simulink model "backstepping"  (R2022b)
settings: Solver=VariableStepAuto  StartTime=0.0  StopTime=30.0  RelTol=1e-3
values from neighbouring files (symbols this model uses):
  Lamda = 10*eye(3)    [init.m]
settings Model: Creator=alexi  LastModifiedBy=alexi

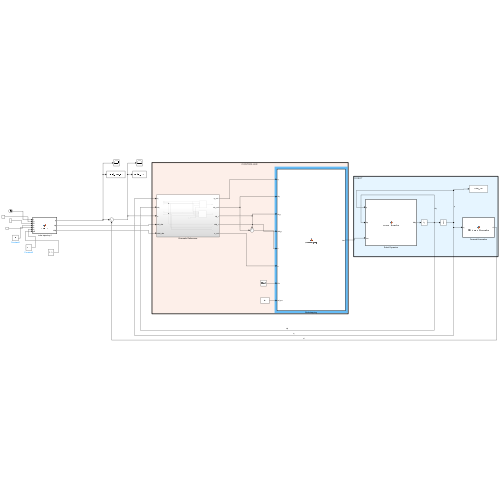
[thumbnail: Simulink's stored preview of the top-level diagram]
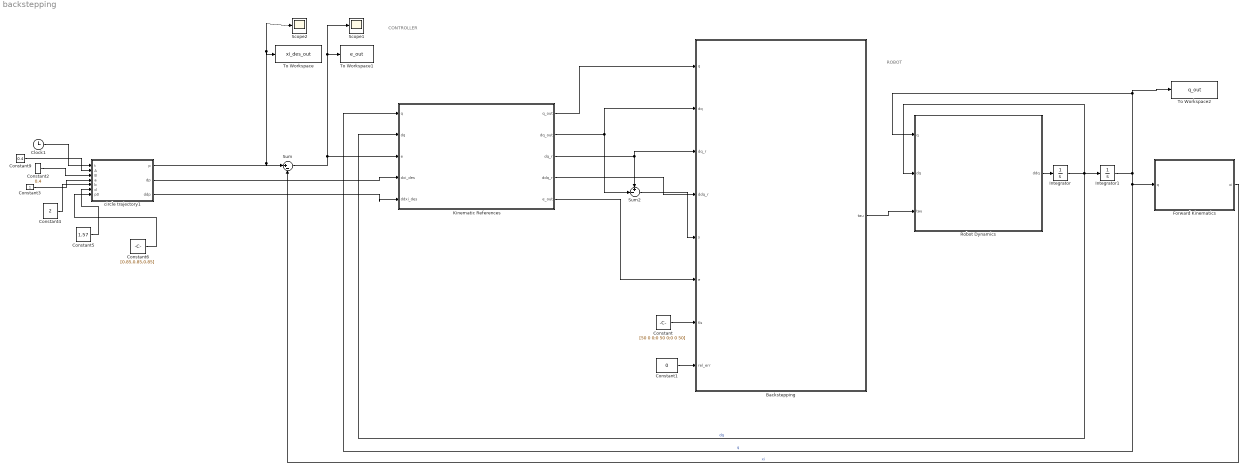
== system backstepping ==
  note: CONTROLLER
  note: ROBOT
  Backstepping : MATLAB Function  TreatAsAtomicUnit=on
  Clock1 : Clock
  Constant : Constant  Value=[50 0 0;0 50 0;0 0 50]
  Constant1 : Constant  Value=0
  Constant2 : Constant  Value=0.4
  Constant3 : Constant
  Constant4 : Constant  Value=2
  Constant5 : Constant  Value=1.57
  Constant6 : Constant  Value=[0.85,0.85,0.85]
  Constant9 : Constant  Value=0.4
  Forward Kinematics : MATLAB Function  TreatAsAtomicUnit=on
  Integrator : Integrator  InitialCondition=[0,0,0]'
  Integrator1 : Integrator  InitialCondition=[0.25,0.25,0.25]'
  Kinematic References : Subsystem
  Robot Dynamics : MATLAB Function  TreatAsAtomicUnit=on
  Scope1 : Scope
  Scope2 : Scope
  Sum : Sum  Inputs=|+-
  Sum2 : Sum  Inputs=+-|
  To Workspace : ToWorkspace  VariableName=xi_des_out  SaveFormat=Timeseries  SampleTime=-1
  To Workspace1 : ToWorkspace  VariableName=e_out  SaveFormat=Timeseries  SampleTime=-1
  To Workspace2 : ToWorkspace  VariableName=q_out  SaveFormat=Timeseries  SampleTime=-1
  circle trajectory1 : MATLAB Function  TreatAsAtomicUnit=on
  wires:
  Kinematic References/4(ddq_r) -> Backstepping/4(ddq_r)
  circle trajectory1/1(p) -> Scope2/1, To Workspace/1, Sum/1
  Kinematic References/2(dq_out) -> Sum2/2, Backstepping/2(dq)
  Sum2/1 -> Backstepping/5(s)
  circle trajectory1/3(ddp) -> Kinematic References/5(ddxi_des)
  Constant/1 -> Backstepping/7(Ks)
  Forward Kinematics/1(xi) -> Sum/2  "xi"
  Kinematic References/1("q_out ") -> Backstepping/1(q)
  Integrator/1 -> Robot Dynamics/2(dq), Kinematic References/2(dq), Integrator1/1  "dq"
  Sum/1 -> Kinematic References/3(e), To Workspace1/1, Scope1/1
  Integrator1/1 -> Kinematic References/1(q), Forward Kinematics/1(q), To Workspace2/1, Robot Dynamics/1(q)  "q"
  circle trajectory1/2(dp) -> Kinematic References/4(dxi_des)
  Backstepping/1(tau) -> Robot Dynamics/3(tau)
  Robot Dynamics/1(ddq) -> Integrator/1
  Kinematic References/3(dq_r) -> Backstepping/3(dq_r), Sum2/1
  Kinematic References/5(e_out) -> Backstepping/6(e)
  Clock1/1 -> circle trajectory1/1(t)
  Constant1/1 -> Backstepping/8(rel_err)
  Constant9/1 -> circle trajectory1/2(A)
  Constant2/1 -> circle trajectory1/3(B)
  Constant3/1 -> circle trajectory1/4(a)
  Constant4/1 -> circle trajectory1/5(b)
  Constant5/1 -> circle trajectory1/6(d)
  Constant6/1 -> circle trajectory1/7(p0)

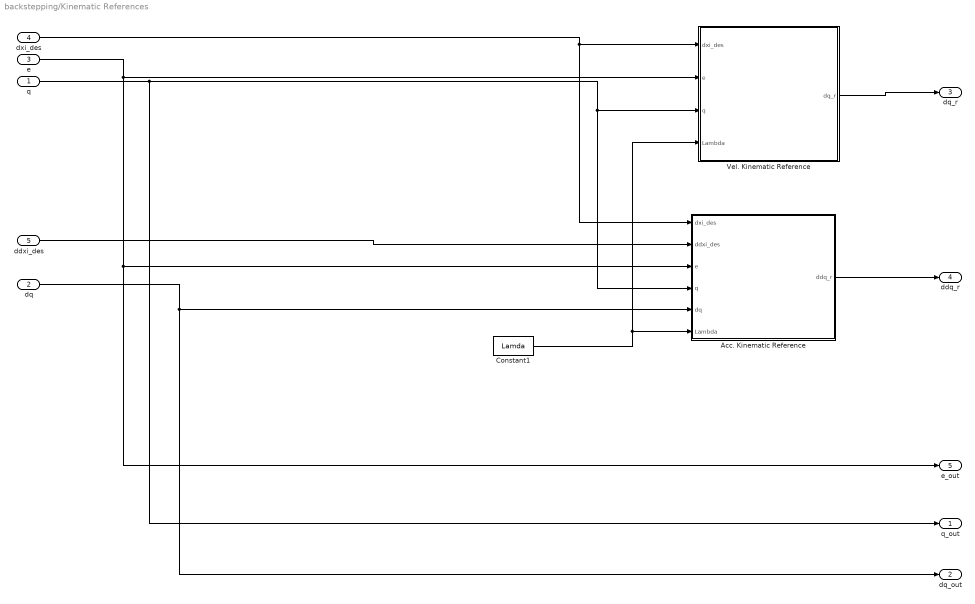
== system backstepping/Kinematic References ==
  q : Inport
  dq : Inport  Port=2
  e : Inport  Port=3
  dxi_des : Inport  Port=4
  ddxi_des : Inport  Port=5
  Acc. Kinematic Reference : MATLAB Function  TreatAsAtomicUnit=on
  Constant1 : Constant  Value=Lamda
  "Vel. Kinematic Reference " : MATLAB Function  TreatAsAtomicUnit=on
  "q_out " : Outport  VectorParamsAs1DForOutWhenUnconnected=off
  dq_out : Outport  Port=2  VectorParamsAs1DForOutWhenUnconnected=off
  dq_r : Outport  Port=3  VectorParamsAs1DForOutWhenUnconnected=off
  ddq_r : Outport  Port=4  VectorParamsAs1DForOutWhenUnconnected=off
  e_out : Outport  Port=5  VectorParamsAs1DForOutWhenUnconnected=off
  wires:
  ddxi_des/1 -> Acc. Kinematic Reference/2(ddxi_des)
  e/1 -> e_out/1, Acc. Kinematic Reference/3(e), "Vel. Kinematic Reference "/2(e)
  dxi_des/1 -> Acc. Kinematic Reference/1(dxi_des), "Vel. Kinematic Reference "/1(dxi_des)
  Constant1/1 -> "Vel. Kinematic Reference "/4(Lambda), Acc. Kinematic Reference/6(Lambda)
  "Vel. Kinematic Reference "/1(dq_r) -> dq_r/1
  dq/1 -> dq_out/1, Acc. Kinematic Reference/5(dq)
  q/1 -> "q_out "/1, Acc. Kinematic Reference/4(q), "Vel. Kinematic Reference "/3(q)
  Acc. Kinematic Reference/1(ddq_r) -> ddq_r/1

== matlab function backstepping/Kinematic References/Acc. Kinematic Reference ==
  data: dxi_des input; ddq_r output; ddxi_des input; e input; q input; dq input; Lambda input
function ddq_r = acc_kinematic_reference(dxi_des, ddxi_des, e, q, dq, Lambda)

coder.extrinsic('disp');

J = zeros(3,3);
dJ = zeros(3,3);

dq1 = dq(1);
dq2 = dq(2);
dq3 = dq(3);

q1 = q(1);
q2 = q(2);
q3 = q(3);

a1 = 1;
a2 = 1;
a3 = 1;

% Computing jacobian and derivative
J = [- a1*sin(q1) - a3*cos(q3)*(cos(q1)*sin(q2) + cos(q2)*sin(q1)) - a2*cos(q1)*sin(q2) - a2*cos(q2)*sin(q1), -a3*cos(q3)*(cos(q1)*sin(q2) +cos(q2)*sin(q1)) - a2*cos(q1)*sin(q2) - a2*cos(q2)*sin(q1), -a3*sin(q3)*(cos(q1)*cos(q2) - sin(q1)*sin(q2)); ...
    a1*cos(q1) + a3*cos(q3)*(cos(q1)*cos(q2) - sin(q1)*sin(q2)) + a2*cos(q1)*cos(q2) - a2*sin(q1)*sin(q2),   a3*cos(q3)*(cos(q1)*cos(q2) - sin(q1)*sin(q2)) + a2*cos(q1)*cos(q2) - a2*sin(q1)*sin(q2),  -a3*sin(q3)*(cos(q1)*sin(q2) + cos(q2)*sin(q1)); ...
    0,0,- a3*cos(q3)*(cos(q1)*sin(q2) + cos(q2)*sin(q1))^2 - a3*cos(q3)*(cos(q1)*cos(q2) - sin(q1)*sin(q2))^2];

a11 = -a1*dq1*cos(q1)-a3*(dq1*cos(q1+q2)+ dq2*cos(q1+q2))*sin(q3)-a2*(dq1*cos(q1+q2)+ dq2*cos(q1+q2));
a12 = -a3*( dq1*cos(q1+q2)+ dq2*cos(q1+q2))*sin(q3)-a2*( dq1*cos(q1+q2)+ dq2*cos(q1+q2));
a13 = -a3*( dq1*cos(q1+q2)+ dq2*cos(q1+q2))*cos(q3);
a21 = -a1*dq1*sin(q1)-a3*( dq1*sin(q1+q2)+ dq2*sin(q1+q2))*cos(q3)-a2*( dq1*sin(q1+q2)+ dq2*sin(q1+q2));
a22 = -a3*(dq1*sin(q1+q2)+dq2*sin(q1+q2))*sin(q3)-a2*(dq1*sin(q1+q2)+dq2*sin(q1+q2));
a23 = -a3*(dq1*cos(q1+q2)+dq2*cos(q1+q2))*sin(q3);
a31 = 0;
a32 = 0;
a33 = 2*a3*(dq1*cos(q1+q2)+dq2*cos(q1+q2))*sin(q1+q2)*sin(q3)-2*a3*(dq1*sin(q1+q2)+dq2*sin(q1+q2))*cos(q1+q2)*sin(q3);

dJ = [a11,a12,a13;a21,a22,a23;a31,a32,a33];

ddq_r = inv(J) * (ddxi_des + Lambda*dxi_des - Lambda*J*dq) ...
- inv(J)*dJ*inv(J)*(dxi_des + Lambda*e);
end

== matlab function backstepping/circle trajectory1 ==
  data: t input; p output; dp output; ddp output; A input; B input; a input; b input; d input; p0 input
function [p,dp,ddp] = lissajous(t,A,B,a,b,d,p0)
C = 0.1;  % Ampiezza dell'oscillazione in z
c = 0.2;  % Frequenza in z
phi = pi/4;
p = [A*sin(a*t+d); B*sin(b*t);C*sin(c*t + phi)] + p0;
dp = [A*a*cos(a*t+d); B*b*cos(b*t);C*c*cos(c*t+phi)];
ddp = [-A*a^2*sin(a*t+d); -B*b^2*sin(b*t);-C*c^2*sin(c*t+phi)];
% a = 0.2;    % Ampiezza lungo l'asse X
% b = 0.2;    % Ampiezza lungo l'asse Y
% p0 = [1;0.8;0.8];
% 
% x = a * cos(t);
% y = b * sin(t);
% z =  0.1 * sin(t);
% 
% p = [x y z]'+p0;
% 
% dx = -a*sin(t);
% dy = b*cos(t);
% dz = 0.5*cos(t);
% 
% dp = [dx dy dz]';
% 
% ddx = -a*cos(t);
% ddy = -b*sin(t);
% ddz = -0.5*sin(t);
% 
% ddp = [ddx ddy ddz]';

== matlab function backstepping/Kinematic References/Vel. Kinematic Reference  ==
  data: dxi_des input; dq_r output; e input; q input; Lambda input
function dq_r = vel_kinematic_reference(dxi_des, e, q, Lambda)
a1 = 1;
a2 = 1;
a3 = 1;

q1 = q(1);
q2 = q(2);
q3 = q(3);

% Computing jacobian
J = [- a1*sin(q1) - a3*cos(q3)*(cos(q1)*sin(q2) + cos(q2)*sin(q1)) - a2*cos(q1)*sin(q2) - a2*cos(q2)*sin(q1), -a3*cos(q3)*(cos(q1)*sin(q2) +cos(q2)*sin(q1)) - a2*cos(q1)*sin(q2) - a2*cos(q2)*sin(q1), -a3*sin(q3)*(cos(q1)*cos(q2) - sin(q1)*sin(q2)); ...
    a1*cos(q1) + a3*cos(q3)*(cos(q1)*cos(q2) - sin(q1)*sin(q2)) + a2*cos(q1)*cos(q2) - a2*sin(q1)*sin(q2),   a3*cos(q3)*(cos(q1)*cos(q2) - sin(q1)*sin(q2)) + a2*cos(q1)*cos(q2) - a2*sin(q1)*sin(q2),  -a3*sin(q3)*(cos(q1)*sin(q2) + cos(q2)*sin(q1)); ...
    0,0,- a3*cos(q3)*(cos(q1)*sin(q2) + cos(q2)*sin(q1))^2 - a3*cos(q3)*(cos(q1)*cos(q2) - sin(q1)*sin(q2))^2];

dq_r = inv(J) * (dxi_des + Lambda*e);
end

== matlab function backstepping/Backstepping ==
  data: q input; dq input; dq_r input; ddq_r input; s input; e input; Ks input; rel_err input; tau output
function tau = backstepping(q, dq, dq_r, ddq_r, s, e, Ks, rel_err)

coder.extrinsic('disp');

% Get dynamic matrices
B = RRR_mass_matrix(q);
C = RRR_coriolis_matrix(q,dq);
G = RRR_gravity_matrix(q);

% Adding uncertainty
B = B.*(1 + rel_err);
C = C.*(1 + rel_err);
G = G.*(1 + rel_err);

a1 = 1;
a2 = 1;
a3 = 1;
q1 = q(1);
q2 = q(2);
q3 = q(3);
% Get Jacobian
J = [- a1*sin(q1) - a3*cos(q3)*(sin(q1+q2)) - a2*sin(q1+q2), -a3*cos(q3)*(sin(q1+q2)) - a2*sin(q1+q2), -a3*sin(q3)*(cos(q1+q2)); ...
    a1*cos(q1) + a3*cos(q3)*(cos(q1+q2)) + a2*cos(q1+q2),   a3*cos(q3)*(cos(q1+q2)) + a2*cos(q1+q2),  -a3*sin(q3)*(sin(q1+q2)); ...
    0,0,- a3*cos(q3)*(sin(q1+q2))^2 - a3*cos(q3)*(cos(q1+q2))^2];

% Control law
tau = B*ddq_r + C*dq_r + G + Ks*s + J.'*e;

== matlab function backstepping/Robot Dynamics ==
  data: q input; dq input; tau input; ddq output
function ddq = inverse_dynamics(q, dq, tau)

% Get dynamic matrices
B = RRR_mass_matrix(q);
C = RRR_coriolis_matrix(q,dq);
G = RRR_gravity_matrix(q);
ddq = pinv(B)*(tau - C*dq - G);

== matlab function backstepping/Forward Kinematics ==
  data: q input; xi output
function xi  = RR_forward_kinematics(q)

    q1 = q(1);
    q2 = q(2);
    q3 = q(3);

    a1 = 1;
    a2 = 1;
    a3 = 1;

    p0 = [0;0;0];
    p1 = [a1*cos(q1); a1*sin(q1);0];
    p2 = p1+[a2*cos(q1+q2);a2*sin(a1+q2);0];
    xi = [a1*cos(q1) + a3*cos(q3)*(cos(q1)*cos(q2) - sin(q1)*sin(q2)) + a2*cos(q1)*cos(q2) - a2*sin(q1)*sin(q2); a1*sin(q1) + a3*cos(q3)*(cos(q1)*sin(q2) + cos(q2)*sin(q1)) + a2*cos(q1)*sin(q2) + a2*cos(q2)*sin(q1);-a3*sin(q3)];
end
